simulink model "P_O_Algorithm"  (R2018a)
settings: Solver=ode23t  StartTime=0.0  StopTime=5  RelTol=1e-3
undefined symbols (not defined in the file): Ion, Lithium
libraries: powerlib x6, electricdrivelib x1, re_lib x1, simulink x1
settings Model: Creator=soura  LastModifiedBy=soura

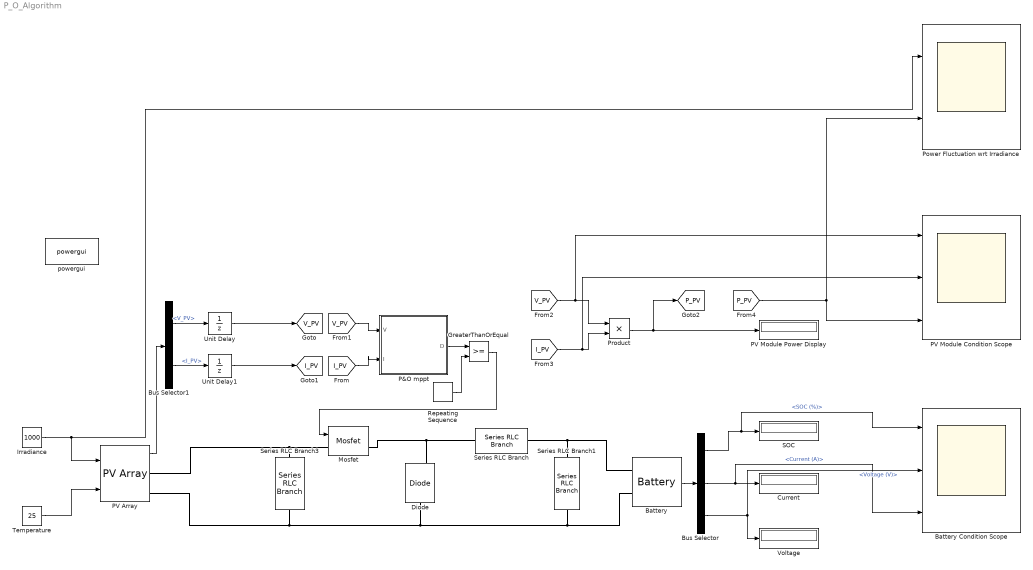
== system P_O_Algorithm ==
  Battery : electricdrivelib/Extra Sources/Battery  BatType=Lithium-Ion  ShowTempParam=off  ThermalPreset=no  ShowAgeParam=off  NomV=12  NomQ=2.5  SOC=20  Batt_Tr=0.01  PresetModel=on  MaxQ=2.5  MinV=9  FullV=13.9678  Dis_rate=1.087  R=0.048  Normal_OP=2.2609  expZone="[12.9646     0.122826]"  current=[6.5 13 32.5]  Units=Time  Tci=20  NomT=20  T2=-30  MaxQ2=4.8  FullV2=7.1  Normal_OP2=5.655  expZone2="[6.58           1]"  Rca=0.6  ti=2000  Dp=0  Neq0=0  Tsim=1e6  Ta1=25  Qeol=5.4*0.9  Reol=0.013333*1.2  Char_age=[2.3478, 3]  Dis_age=[2.3478, 10]  N1=1500  N2=10500  N3=1000  N4=1400  Ta2=45  N5=950
  Battery Condition Scope : Scope  NumInputPorts=3
  Bus Selector : BusSelector  OutputSignals=SOC (%),Current (A),Voltage (V)
  Bus Selector1 : BusSelector  OutputSignals=V_PV,I_PV
  Current : Display
  Diode : powerlib/Power Electronics/Diode  Ron=0.001  Lon=0  Vf=0.8  IC=0  UseSnubber=0  Rs=500  Cs=250e-9  Measurements=on
  GreaterThanOrEqual : RelationalOperator  OutDataTypeStr=boolean  RndMeth=Simplest
  Irradiance : Constant  Value=1000
  Mosfet : powerlib/Power Electronics/Mosfet  Ron=0.1  Lon=0  Rd=0.01  Vfd=0  IC=0  Rs=1e5  Cs=inf  Measurements=on
  "P&O mppt " : MATLAB Function  TreatAsAtomicUnit=on
  PV Array : re_lib/Solar/PV Array  Npar=1  Nser=1  PlotType=one module @ 25 deg.C & specified irradiances  S_vec="[ 1000  500  100 ]"  Temp_C_vec="[ 45 25  ]"  ModuleName=User-defined  PlotWhenSelected=off  Pm=213.15  Ncell=60  Voc=36.3  Isc=7.84  Vm=29  Im=7.35  beta_Voc_pc=-0.36099  alpha_Isc_pc=0.102  beta_Voc=-0.13104  alpha_Isc=0.0079968  IL=7.8654  I0=2.9273e-10  nI=0.98119  Rsh=313.0553  Rs=0.39381  BAL=on  Tc=1e-6  Tfilter=5e-5
  PV Module Condition Scope : Scope  NumInputPorts=3
  PV Module Power Display : Display
  Power Fluctuation wrt Irradiance : Scope  NumInputPorts=2
  Product : Product
  Repeating Sequence : simulink/Sources/Repeating Sequence  rep_seq_t=[0 0.0002]  rep_seq_y=[0 1]
  SOC : Display
  Series RLC Branch : powerlib/Elements/Series RLC Branch  LConnTagsString=__new0  RConnTagsString=__new0  BranchType=L  Resistance=1  Inductance=0.8653e-3  SetiL0=off  InitialCurrent=0  Capacitance=1e-6  Setx0=off  InitialVoltage=0  Measurements=None
  Series RLC Branch1 : powerlib/Elements/Series RLC Branch  LConnTagsString=__new0  RConnTagsString=__new0  BranchType=C  Resistance=1  Inductance=1e-3  SetiL0=off  InitialCurrent=0  Capacitance=369.79e-6  Setx0=off  InitialVoltage=0  Measurements=None
  Series RLC Branch3 : powerlib/Elements/Series RLC Branch  LConnTagsString=__new0  RConnTagsString=__new0  BranchType=RC  Resistance=0.001  Inductance=1e-3  SetiL0=off  InitialCurrent=0  Capacitance=1000e-6  Setx0=off  InitialVoltage=0  Measurements=None
  "Temperature " : Constant  Value=25
  Unit Delay : UnitDelay  SampleTime=1e-4
  Unit Delay1 : UnitDelay  SampleTime=1e-4
  Voltage : Display
  powergui : powerlib/powergui  Priority=1  SimulationMode=Discrete  SampleTime=1e-06  frequency=60  Iterations=50  frequencyindice=0  Pbase=100e6  ErrMax=1e-4  UnitsV=kV  UnitsW=MW  buscounter=0  FunctionMessages=off  echomessages=off  EnableUseOfTLC=off  CurrentSourceSwitches=off  DisableSnubberDevices=off  DisableRonSwitches=off  DisableVfSwitches=off  DisplayEquations=off  SolverType=Tustin/Backward Euler (TBE)  Interpol=off  ExternalGateDelay=off  methode=off  Ts=100  x0status=blocks  SPID=on  SwTol=0  HookPort=off  RestoreLinks=warning  ResistiveCurrentMeasurement=off  Frange=[0:2:500]  Ylog=off  Xlog=on  ShowGrid=off  save=off  variable=ZData  structure=0  ZoomFFT=off  StartTime=0.0  cycles=1  DisplayStyle=1  fundamental=60  FreqAxis=off  MaxFrequency=1000  frequencyindicesteady=1  RmsSteady=1  display=off
  tag scope: I_PV=global, P_PV=global, V_PV=global
  wires:
  "Temperature "/1 -> PV Array/2
  [V_PV] -> PV Module Condition Scope/1, Product/1
  [I_PV] -> "P&O mppt "/2(I)
  GreaterThanOrEqual/1 -> Mosfet/1
  Unit Delay/1 -> [V_PV]
  Bus Selector1/1 -> Unit Delay/1  "<V_PV>"
  Bus Selector/3 -> Voltage/1, Battery Condition Scope/2  "<Voltage (V)>"
  Bus Selector/2 -> Battery Condition Scope/3, Current/1  "<Current (A)>"
  "P&O mppt "/1(D) -> GreaterThanOrEqual/1
  PV Array/1 -> Bus Selector1/1
  Product/1 -> [P_PV], PV Module Power Display/1
  Repeating Sequence/1 -> GreaterThanOrEqual/2
  Irradiance/1 -> Power Fluctuation wrt Irradiance/1, PV Array/1
  Battery/1 -> Bus Selector/1
  Unit Delay1/1 -> [I_PV]
  Bus Selector1/2 -> Unit Delay1/1  "<I_PV>"
  [V_PV] -> "P&O mppt "/1(V)
  [I_PV] -> PV Module Condition Scope/2, Product/2
  Bus Selector/1 -> Battery Condition Scope/1, SOC/1  "<SOC (%)>"
  [P_PV] -> Power Fluctuation wrt Irradiance/2, PV Module Condition Scope/3
  connections:
  PV Array/RConn1 -- Series RLC Branch3/LConn1 -- Mosfet/LConn1
  Series RLC Branch1/LConn1 -- Battery/LConn1 -- Series RLC Branch/RConn1
  Series RLC Branch1/RConn1 -- Diode/LConn1 -- Series RLC Branch3/RConn1 -- PV Array/RConn2 -- Battery/LConn2
  Diode/RConn1 -- Series RLC Branch/LConn1 -- Mosfet/RConn1

== matlab function P_O_Algorithm/P&O mppt  ==
  data: V input; D output; I input
function D = Duty_Cycle(V,I)
Dmax = 0.95;
Dmin = 0;
Dinit = 0.95;
De1D = 0.0001;
persistent Vo1d Po1d Do1d;

datatype = 'double' ;

if isempty(Vo1d)
    Vo1d = 0;
    Po1d = 0;
    Do1d = Dinit;
end

P = V * I;
dV = V-Vo1d;
dP = P-Po1d;
if dP ~= 0
    if dP < 0
        if dV < 0
            D = Do1d - De1D;
        else
            D = Do1d + De1D;
        end
    else
        if dV < 0
            D = Do1d + De1D;
        else
            D = Do1d - De1D;
        end
     end
else
        D = Do1d;
end

if D >= Dmax || D < Dmin
    D = Do1d;
end
Vo1d = V;
Po1d = P;
Do1d = D;
end
